simulink model "rascunho_LS"  (Simulink 10.3)
settings: Solver=VariableStepAuto  StartTime=0.0  StopTime=10.0  RelTol=1e-3
values from neighbouring files (symbols this model uses):
  As = 2    [sim_grad_norm.m]    (also in sim_grad_norm_3ordem.m = 0)
  DC = 1    [sim_grad_norm.m]    (also in sim_grad_norm_3ordem.m)
  kappa = 1e-9    (= 1e-09)    [sim_grad_norm.m]    (also in sim_grad_norm_3ordem.m = 1)
  lambda0 = 1    [sim_grad_norm.m]    (also in sim_grad_norm_3ordem.m)
  lambda1 = 2    [sim_grad_norm.m]    (also in sim_grad_norm_3ordem.m)
  lambda2 = 3    [sim_grad_norm.m]    (also in sim_grad_norm_3ordem.m)
  P0 = eye(6)    [sim_grad_norm.m]    (also in sim_grad_norm_3ordem.m = 1*eye(6))
  st = 0.01    [sim_grad_norm.m]    (also in sim_grad_norm_3ordem.m)
  theta0 = [0;0;0;0;0;0]    [sim_grad_norm.m]    (also in sim_grad_norm_3ordem.m)
  theta_star = theta_star3    [sim_grad_norm.m]    (also in sim_grad_norm_3ordem.m = theta_star1)
  ws = 0.1*pi    (= 0.314159265359)    [sim_grad_norm.m]    (also in sim_grad_norm_3ordem.m = 3.14159265359)
libraries: cstblocks x1
settings Model: Creator=caioc  LastModifiedBy=caioc
settings SolverCC: AlgebraicLoopSolver=Auto
settings DataIOCC: SaveFormat=Dataset  SignalLoggingSaveFormat=Dataset  ReturnWorkspaceOutputs=on
settings OptimizationCC: ExpressionDepthLimit=128  LifeSpan=auto
settings DebuggingCC: UnderspecifiedInitializationDetection=Simplified  MergeDetectMultiDrivingBlocksExec=error  FcnCallInpInsideContextMsg=error  StateNameClashWarn=none  SFUnexpectedBacktrackingDiag=error  SFNoUnconditionalDefaultTransitionDiag=error  SFExecutionAtInitializationDiag=warning  SFMachineParentedDataDiag=error  ArithmeticOperatorsInVariantConditions=error
settings HardwareCC: ProdBitPerPointer=64  ProdBitPerSizeT=64  ProdBitPerPtrDiffT=64  ProdLargestAtomicFloat=Float  ProdIntDivRoundTo=Zero  ProdEndianess=LittleEndian  ProdWordSize=64  ProdHWDeviceType=Intel->x86-64 (Windows64)
settings ModelReferenceCC: PropagateSignalLabelsOutOfModel=on
settings SFSimCC: SimUseLocalCustomCode=on  CustomCodeUndefinedFunction=FilterOut
settings RTWCC: RTWUseLocalCustomCode=on
settings CodeAppCC: StateflowObjectComments=off
settings GRTTargetCC: TargetLangStandard=C99 (ISO)  CombineOutputUpdateFcns=on  GRTInterface=off
settings ConfigComp: CovMetricSettings=dwe  CovSaveCumulativeToWorkspaceVar=off  CovSaveSingleToWorkspaceVar=off  CovExternalEMLEnable=on

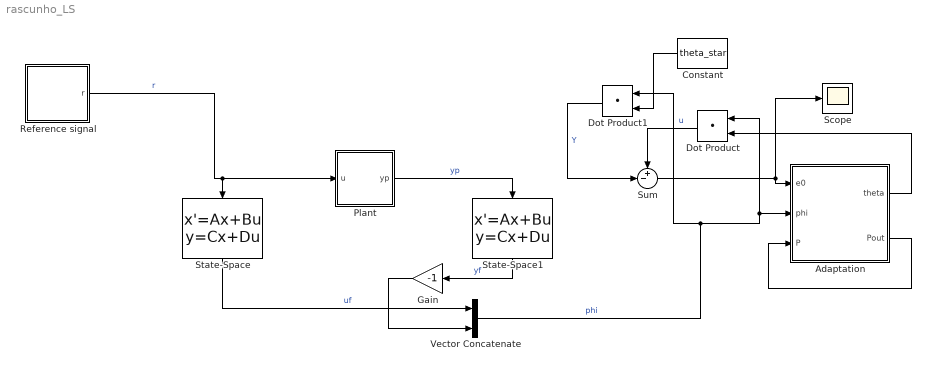
== system rascunho_LS ==
  Adaptation : Subsystem
  Constant : Constant  Value=theta_star
  Dot Product : DotProduct  InputSameDT=on  OutDataTypeStr=Inherit: Inherit via internal rule
  Dot Product1 : DotProduct  InputSameDT=on  OutDataTypeStr=Inherit: Inherit via internal rule
  Gain : Gain  Gain=-1
  Plant : Subsystem
  Reference signal : Subsystem
  Scope : Scope
  State-Space : StateSpace  A=[0 1 0;0 0 1; -lambda0 -lambda1 -lambda2]  B=[0; 0; 1]  C=[1 0 0;0 1 0; 0 0 1]  D=[0;0;0]  InitialCondition=0
  State-Space1 : StateSpace  A=[0 1 0;0 0 1; -lambda0 -lambda1 -lambda2]  B=[0; 0; 1]  C=[1 0 0;0 1 0; 0 0 1]  D=[0;0;0]  InitialCondition=0
  Sum : Sum  Inputs=+-|
  Vector Concatenate : Concatenate
  wires:
  Dot Product1/1 -> Sum/2  "Y"
  Constant/1 -> Dot Product1/2
  State-Space1/1 -> Gain/1  "yf"
  Sum/1 -> Scope/1, Adaptation/1(e0)
  Gain/1 -> Vector Concatenate/2
  Reference signal/1(r) -> State-Space/1, Plant/1(u)  "r"
  Vector Concatenate/1 -> Dot Product/1, Adaptation/2(phi), Dot Product1/1  "phi"
  Plant/1(yp) -> State-Space1/1  "yp"
  Adaptation/1(theta) -> Dot Product/2
  State-Space/1 -> Vector Concatenate/1  "uf"
  Dot Product/1 -> Sum/1  "u"
  Adaptation/2(Pout) -> Adaptation/3(P)

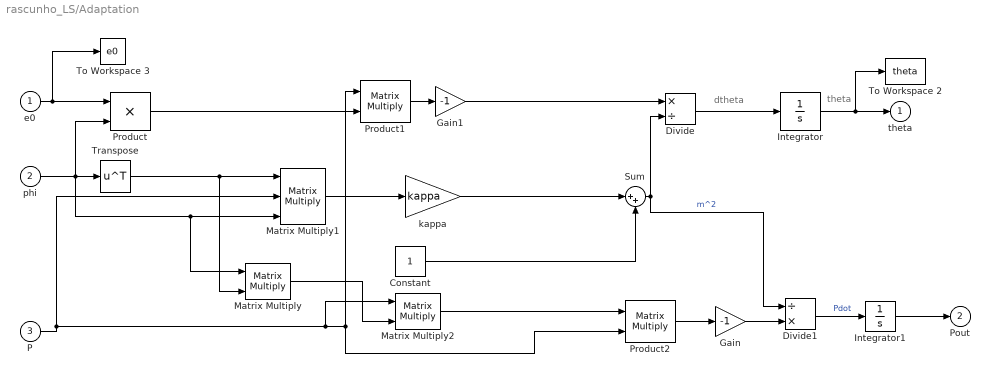
== system rascunho_LS/Adaptation ==
  note: theta
  note: dtheta
  e0 : Inport  PortDimensions=1
  phi : Inport  Port=2
  P : Inport  Port=3
  Constant : Constant
  Divide : Product  Inputs=*/
  Divide1 : Product  Inputs=/*
  Gain : Gain  Gain=-1
  Gain1 : Gain  Gain=-1
  Integrator : Integrator  InitialCondition=theta0
  Integrator1 : Integrator  InitialCondition=P0
  Matrix Multiply : Product  Multiplication=Matrix(*)
  Matrix Multiply1 : Product  Inputs=3  Multiplication=Matrix(*)
  Matrix Multiply2 : Product  Multiplication=Matrix(*)
  Product : Product  InputSameDT=on  RndMeth=Zero  SaturateOnIntegerOverflow=on  OutDataTypeStr=Inherit: Same as first input
  Product1 : Product  Multiplication=Matrix(*)
  Product2 : Product  Multiplication=Matrix(*)
  Sum : Sum  Inputs=|++
  To Workspace 2 : ToWorkspace  VariableName=theta  SampleTime=st
  To Workspace 3 : ToWorkspace  VariableName=e0  SampleTime=st
  Transpose : Math  Operator=transpose  SaturateOnIntegerOverflow=on
  kappa : Gain  Gain=kappa  SaturateOnIntegerOverflow=on  OutDataTypeStr=Inherit: Same as input  ParamDataTypeStr=Inherit: Same as input
  theta : Outport  InitialOutput=0  VectorParamsAs1DForOutWhenUnconnected=off
  Pout : Outport  Port=2  InitialOutput=0  VectorParamsAs1DForOutWhenUnconnected=off
  wires:
  Integrator/1 -> To Workspace 2/1, theta/1
  Divide/1 -> Integrator/1
  e0/1 -> Product/1, To Workspace 3/1
  Product1/1 -> Gain1/1
  Product/1 -> Product1/2
  phi/1 -> Matrix Multiply/1, Matrix Multiply1/3, Transpose/1, Product/2
  Constant/1 -> Sum/2
  kappa/1 -> Sum/1
  Sum/1 -> Divide1/1, Divide/2  "m^2"
  P/1 -> Matrix Multiply2/1, Product2/2, Product1/1, Matrix Multiply1/2
  Product2/1 -> Gain/1
  Matrix Multiply/1 -> Matrix Multiply2/2
  Transpose/1 -> Matrix Multiply1/1, Matrix Multiply/2
  Matrix Multiply1/1 -> kappa/1
  Integrator1/1 -> Pout/1
  Gain1/1 -> Divide/1
  Matrix Multiply2/1 -> Product2/1
  Gain/1 -> Divide1/2
  Divide1/1 -> Integrator1/1  "Pdot"

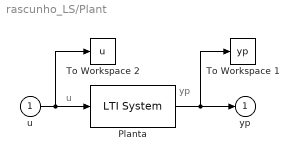
== system rascunho_LS/Plant ==
  note: yp
  note: u
  u : Inport
  Planta : cstblocks/LTI System  sys=P  IC=x0
  To Workspace 1 : ToWorkspace  VariableName=yp  SampleTime=st
  To Workspace 2 : ToWorkspace  VariableName=u  SampleTime=st
  yp : Outport  InitialOutput=0  VectorParamsAs1DForOutWhenUnconnected=off
  wires:
  u/1 -> To Workspace 2/1, Planta/1
  Planta/1 -> yp/1, To Workspace 1/1

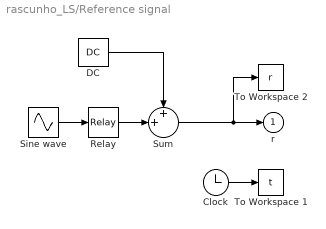
== system rascunho_LS/Reference signal ==
  Clock : Clock
  DC : Constant  Value=DC
  Relay : Relay  OnOutputValue=As  OffOutputValue=-As
  Sine wave : Sin  Frequency=ws  SampleTime=0
  Sum : Sum  Inputs=++|  InputSameDT=on  SaturateOnIntegerOverflow=on  OutDataTypeStr=Inherit: Same as first input
  To Workspace 1 : ToWorkspace  VariableName=t  SampleTime=st
  To Workspace 2 : ToWorkspace  VariableName=r  SampleTime=st
  r : Outport  InitialOutput=0  VectorParamsAs1DForOutWhenUnconnected=off
  wires:
  DC/1 -> Sum/1
  Sum/1 -> r/1, To Workspace 2/1
  Clock/1 -> To Workspace 1/1
  Sine wave/1 -> Relay/1
  Relay/1 -> Sum/2
